simulink model "Control_Lyapunov_BarcoDiferencial"  (R2022a)
settings: Solver=VariableStepAuto  StartTime=0.0  StopTime=600  RelTol=1e-3
libraries: robotcorelib x3
settings Model: Creator=Lenovo  LastModifiedBy=Lenovo

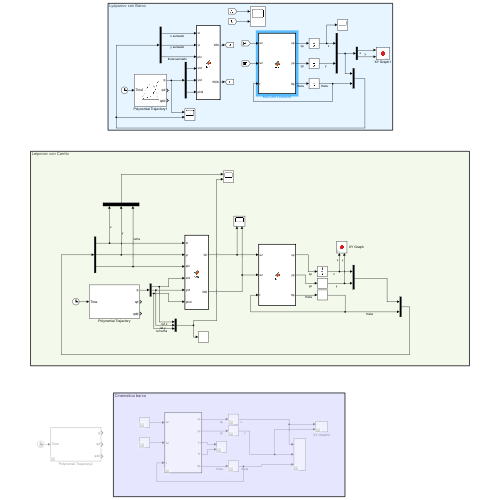
[thumbnail: Simulink's stored preview of the top-level diagram]
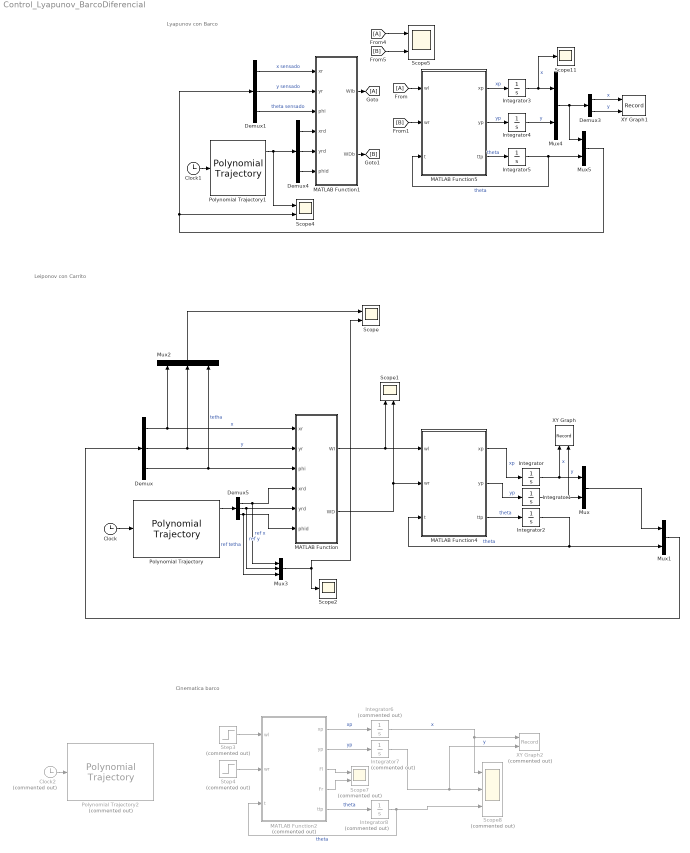
== system Control_Lyapunov_BarcoDiferencial ==
  note: Leiponov con Carrito
  note: Lyapunov con Barco
  note: Cinematica barco
  Clock : Clock
  Clock1 : Clock
  Clock2 : Clock  Commented=on
  Demux{,1,4..5} (4 alike) : Demux  Outputs=3
  Demux3 : Demux  Outputs=2
  From : From
  From4 : From
  Goto : Goto
  Integrator : Integrator  InitialCondition=0.0001
  Integrator1 : Integrator
  Integrator2 : Integrator
  Integrator3 : Integrator  InitialCondition=10
  Integrator4 : Integrator  InitialCondition=5
  Integrator5 : Integrator  InitialCondition=2.7
  Integrator6 : Integrator  Commented=on  InitialCondition=5
  Integrator7 : Integrator  Commented=on  InitialCondition=5
  Integrator8 : Integrator  Commented=on
  MATLAB Function : MATLAB Function  TreatAsAtomicUnit=on
  MATLAB Function1 : MATLAB Function  TreatAsAtomicUnit=on
  MATLAB Function2 : MATLAB Function  Commented=on  TreatAsAtomicUnit=on
  MATLAB Function4 : MATLAB Function  TreatAsAtomicUnit=on
  MATLAB Function5 : MATLAB Function  TreatAsAtomicUnit=on
  Mux{,1,4..5} (4 alike) : Mux  Inputs=2
  Mux2 : Mux  Inputs=3
  Mux3 : Mux  Inputs=3
  Polynomial Trajectory : robotcorelib/Polynomial Trajectory  WaypointSource=Internal  Waypoints=[ 0 5; 0 10; 0 1.578]  TimePoints=[ 0, 50 ]  TimeInterval=[ 1, 4 ]  Method=Cubic Polynomial  ParameterSource=Internal  VelocityBoundaryCondition=zeros( 3, 2)  AccelerationBoundaryCondition=zeros( 2, 5 )  SimulateUsing=Interpreted execution
      settings: SourceProductBaseCode=RO,NV,RR,UV
  Polynomial Trajectory1 : robotcorelib/Polynomial Trajectory  WaypointSource=Internal  Waypoints=[10 12; 5 10; 2.7 1.5]  TimePoints=[0 10]  TimeInterval=[ 1, 4 ]  Method=Cubic Polynomial  ParameterSource=Internal  VelocityBoundaryCondition=zeros( 3, 2)  AccelerationBoundaryCondition=zeros( 2, 5 )  SimulateUsing=Interpreted execution
      settings: SourceProductBaseCode=RO,NV,RR,UV
  Polynomial Trajectory2 : robotcorelib/Polynomial Trajectory  Commented=on  WaypointSource=Internal  Waypoints=[ 0 5; 0 5; 0 1.578]  TimePoints=[ 0 20 ]  TimeInterval=[ 1, 4 ]  Method=Cubic Polynomial  ParameterSource=Internal  VelocityBoundaryCondition=zeros( 3, 2)  AccelerationBoundaryCondition=zeros( 2, 5 )  SimulateUsing=Interpreted execution
      settings: SourceProductBaseCode=RO,NV,RR,UV
  Scope{,1,4..5} (4 alike) : Scope  NumInputPorts=2
  Scope11 : Scope
  Scope2 : Scope
  Scope7 : Scope  Commented=on  NumInputPorts=2
  Scope8 : Scope  Commented=on  NumInputPorts=3
  Step3 : Step  Commented=on  Time=0  After=10  SampleTime=0
  Step4 : Step  Commented=on  Time=0  After=5  SampleTime=0
  XY Graph : Record  FileSettingsInternal="{\"entries\":[{\"content\":{\"excelSettings\":{\"content\":{},\"type\":\"Streamout.ExcelSettings\"}},\"type\":\"Streamout.FileSettingStorage\",\"uuid\":\"7295fb2b-ff57-43ce-bb86-fdd5f6b61bc5\"}],\"packageUris\":[\"http://schema.mathworks.com/mf0/streamout_blocks/R2020a\"],\"version\":\"1.0\"}"  Layout=[1 1]  SignalsInternal="{\"entries\":[{\"content\":{\"signals\":[{\"content\":{\"blockPath\":[\"Diagrma_Base2/XY Graph\"],\"channel\":[],\"dimensions\":[1],\"domain\":\"Diagrma_Base2/XY Graph\",\"lineColor\":\"#a2142f\",\"plots\":[1],\"port\":1,\"sid\":[],\"signalID\":17,\"signalName\":\"x\"},\"type\":\"RecordBlkView.Signal\",\"uuid\":\"777eca82-6aae-4ff1-8555-769b58b9b1a9\"},{\"content\":{\"blockPath\":[\"Diagrma_Base2/XY Graph\"],\"channel\":[],\"dimensions\":[1],\"domain\":\"Diagrma_Base2/XY Graph\",\"lineColor\":\"#139fff\",\"plots\":[1],\"port\":2,\"sid\":[],\"signalID\":20,\"signalName\":\"y\"},\"type\":\"RecordBlkView.Signal\",\"uuid\":\"4820c845-bf9c-47bf-9568-d466896c225b\"}]},\"type\":\"RecordBlkView.InputSignals\",\"uuid\":\"f7904860-0271-4dba-87b7-ce7dfbb5efd7\"}],\"packageUris\":[\"http://schema.mathworks.com/mf0/streamout_blocks/R2020a\"],\"version\":\"1.0\"}"  VisualizationBindings="{\"xyplotplugin\":{\"info\":[{\"series\":[{\"bindingParametersList\":[{\"parameter\":\"X-Axis\",\"signalID\":17,\"signalName\":\"x\"},{\"parameter\":\"Y-Axis\",\"signalID\":20,\"signalName\":\"y\"}],\"seriesID\":12843}],\"subplotID\":1}]}}"  CompatibilityTag=XY
  XY Graph1 : Record  FileSettingsInternal="{\"entries\":[{\"content\":{\"excelSettings\":{\"content\":{},\"type\":\"Streamout.ExcelSettings\"}},\"type\":\"Streamout.FileSettingStorage\",\"uuid\":\"a2b37473-8bde-4ada-a6ad-28720db650b0\"}],\"packageUris\":[\"http://schema.mathworks.com/mf0/streamout_blocks/R2020a\"],\"version\":\"1.0\"}"  Layout=[1 1]  SignalsInternal="{\"entries\":[{\"content\":{\"signals\":[{\"content\":{\"blockPath\":[\"Diagrma_Base2/XY Graph1\"],\"channel\":[],\"dimensions\":[1],\"domain\":\"Diagrma_Base2/XY Graph1\",\"lineColor\":\"#a2142f\",\"plots\":[1],\"port\":1,\"sid\":[],\"signalID\":9,\"signalName\":\"x\"},\"type\":\"RecordBlkView.Signal\",\"uuid\":\"0c049299-8119-4ead-a456-183b3d2d228e\"},{\"content\":{\"blockPath\":[\"Diagrma_Base2/XY Graph1\"],\"channel\":[],\"dimensions\":[1],\"domain\":\"Diagrma_Base2/XY Graph1\",\"lineColor\":\"#139fff\",\"plots\":[1],\"port\":2,\"sid\":[],\"signalID\":12,\"signalName\":\"y\"},\"type\":\"RecordBlkView.Signal\",\"uuid\":\"c17ab7cf-dfc4-43cc-b6cb-2b06547cf23f\"}]},\"type\":\"RecordBlkView.InputSignals\",\"uuid\":\"baae757a-dbf7-4c06-a341-545d20dfedee\"}],\"packageUris\":[\"http://schema.mathworks.com/mf0/streamout_blocks/R2020a\"],\"version\":\"1.0\"}"  VisualizationBindings="{\"xyplotplugin\":{\"info\":[{\"series\":[{\"bindingParametersList\":[{\"parameter\":\"X-Axis\",\"signalID\":9,\"signalName\":\"x\"},{\"parameter\":\"Y-Axis\",\"signalID\":12,\"signalName\":\"y\"}],\"seriesID\":46415}],\"subplotID\":1}]}}"  CompatibilityTag=XY
  XY Graph2 : Record  Commented=on  FileSettingsInternal="{\"entries\":[{\"content\":{\"excelSettings\":{\"content\":{},\"type\":\"Streamout.ExcelSettings\"}},\"type\":\"Streamout.FileSettingStorage\",\"uuid\":\"b3166ed0-6056-44fb-bfad-bac826df8843\"}],\"packageUris\":[\"http://schema.mathworks.com/mf0/streamout_blocks/R2020a\"],\"version\":\"1.0\"}"  Layout=[1 1]  SignalsInternal="{\"entries\":[{\"content\":{\"signals\":[{\"content\":{\"blockPath\":[\"Diagrma_Base2/XY Graph2\"],\"channel\":[],\"dimensions\":[1],\"domain\":\"Diagrma_Base2/XY Graph2\",\"lineColor\":\"#a2142f\",\"plots\":[1],\"port\":1,\"sid\":[],\"signalID\":25,\"signalName\":\"x\"},\"type\":\"RecordBlkView.Signal\",\"uuid\":\"49568a3e-d36f-41cf-8f23-ccc7c9185f6e\"},{\"content\":{\"blockPath\":[\"Diagrma_Base2/XY Graph2\"],\"channel\":[],\"dimensions\":[1],\"domain\":\"Diagrma_Base2/XY Graph2\",\"lineColor\":\"#139fff\",\"plots\":[1],\"port\":2,\"sid\":[],\"signalID\":28,\"signalName\":\"y\"},\"type\":\"RecordBlkView.Signal\",\"uuid\":\"cb959886-84b1-405c-8f57-00818f683079\"}]},\"type\":\"RecordBlkView.InputSignals\",\"uuid\":\"66f7ff6e-8114-4676-a999-c205b5aca1eb\"}],\"packageUris\":[\"http://schema.mathworks.com/mf0/streamout_blocks/R2020a\"],\"version\":\"1.0\"}"  VisualizationBindings="{\"xyplotplugin\":{\"info\":[{\"series\":[{\"bindingParametersList\":[{\"parameter\":\"X-Axis\",\"signalID\":25,\"signalName\":\"x\"},{\"parameter\":\"Y-Axis\",\"signalID\":28,\"signalName\":\"y\"}],\"seriesID\":189}],\"subplotID\":1}]}}"  CompatibilityTag=XY
  wires:
  MATLAB Function/1(WI) -> Scope1/1, MATLAB Function4/1(wl)
  MATLAB Function/2(WD) -> Scope1/2, MATLAB Function4/2(wr)
  MATLAB Function4/1(xp) -> Integrator/1  "xp"
  MATLAB Function4/2(yp) -> Integrator1/1  "yp"
  MATLAB Function4/3(ttp) -> Integrator2/1  "theta"
  Mux/1 -> Mux1/1
  Demux/2 -> Mux2/2, MATLAB Function/2(yr)  "y"
  Mux2/1 -> Scope/1
  Integrator2/1 -> MATLAB Function4/3(t), Mux1/2  "theta"
  Clock/1 -> Polynomial Trajectory/1
  Mux1/1 -> Demux/1
  Integrator1/1 -> XY Graph/2, Mux/2  "y"
  Integrator/1 -> XY Graph/1, Mux/1  "x"
  Mux3/1 -> Scope2/1, Scope/2
  Demux/1 -> Mux2/1, MATLAB Function/1(xr)  "x"
  Demux/3 -> Mux2/3, MATLAB Function/3(phi)  "tetha"
  Mux5/1 -> Scope4/2, Demux1/1
  Demux1/2 -> MATLAB Function1/2(yr)  "y sensado"
  Demux3/1 -> XY Graph1/1  "x"
  Demux1/3 -> MATLAB Function1/3(phi)  "theta sensado"
  Demux1/1 -> MATLAB Function1/1(xr)  "x sensado"
  MATLAB Function5/2(yp) -> Integrator4/1  "yp"
  Integrator5/1 -> MATLAB Function5/3(t), Mux5/2  "theta"
  MATLAB Function5/3(ttp) -> Integrator5/1  "theta"
  Demux3/2 -> XY Graph1/2  "y"
  MATLAB Function5/1(xp) -> Integrator3/1  "xp"
  Integrator4/1 -> Mux4/2  "y"
  Integrator3/1 -> Scope11/1, Mux4/1  "x"
  Mux4/1 -> Demux3/1, Mux5/1
  Clock1/1 -> Polynomial Trajectory1/1
  Demux4/1 -> MATLAB Function1/4(xrd)
  Demux4/3 -> MATLAB Function1/6(phid)
  Demux4/2 -> MATLAB Function1/5(yrd)
  Integrator8/1 -> Scope8/3, MATLAB Function2/3(t)  "theta"
  Integrator6/1 -> XY Graph2/1, Scope8/1  "x"
  MATLAB Function2/5(ttp) -> Integrator8/1  "theta"
  Integrator7/1 -> XY Graph2/2, Scope8/2  "y"
  MATLAB Function2/2(yp) -> Integrator7/1  "yp"
  MATLAB Function2/1(xp) -> Integrator6/1  "xp"
  MATLAB Function2/3(Fl) -> Scope7/1
  MATLAB Function2/4(Fr) -> Scope7/2
  Step4/1 -> MATLAB Function2/2(wr)
  Step3/1 -> MATLAB Function2/1(wl)
  Polynomial Trajectory/1 -> Demux5/1
  Demux5/1 -> MATLAB Function/4(xrd), Mux3/1  "ref x"
  Demux5/2 -> Mux3/2, MATLAB Function/5(yrd)  "ref y"
  Demux5/3 -> MATLAB Function/6(phid), Mux3/3  "ref tetha"
  Clock2/1 -> Polynomial Trajectory2/1
  From4/1 -> Scope5/1
  [B] -> Scope5/2
  MATLAB Function1/1(WIb) -> Goto/1
  From/1 -> MATLAB Function5/1(wl)
  MATLAB Function1/2(WDb) -> [B]
  [B] -> MATLAB Function5/2(wr)
  Polynomial Trajectory1/1 -> Scope4/1, Demux4/1

== matlab function Control_Lyapunov_BarcoDiferencial/MATLAB Function1 ==
  data: xr input; yr input; phi input; xrd input; WIb output; WDb output; yrd input; phid input
function [WIb, WDb]  = fcn(xr, yr, phi, xrd, yrd, phid)
%------------valores barco---------
Lb = 0.87;
Db = 0.435;
K1 = 1;
K2 = 1;
q2 = 1;

% 4) Control
%a) Errores de control
l = sqrt((xrd - xr)^2 + (yrd - yr)^2);
zeta = atan2((yrd - yr), (xrd - xr)) - phi;
psi = atan2((yrd - yr), (xrd - xr)) - phid;
%b) Ley de control
u = K1 * cos(zeta) * l; % Velocidad lineal de entrada
w = K2 * zeta + (K1/zeta) * cos(zeta) * sin(zeta) * (zeta + q2 * psi); % Velocidad angular de entrada

% p -> densidad agua (kg/m^3)
p = 1000;
% r -> radio del motor
r = 0.065;
% A -> Area de la seccion transversal del motor (m^2)
A = (pi*0.065^2);
Fl = p*A*r^2;          % Fuerza de la hélice izquierda (N/s)
Fr = p*A*r^2;          % Fuerza de la hélice derecha (N/s)
%c) velocidades angulares:
% Bote
WDb = Fr*(2*u + Lb*w)/(2*Db);
WIb = Fl*(2*u - Lb*w)/(2*Db);

== matlab function Control_Lyapunov_BarcoDiferencial/MATLAB Function ==
  data: xr input; yr input; phi input; xrd input; WI output; WD output; yrd input; phid input
function [WI, WD]  = fcn(xr, yr, phi, xrd, yrd, phid)
L = 0.87;
D = 0.435;
R = 0.130;
% 2) Condiciones iniciales
% xr, yr, phi

% 3) Referencias deseadas
% xrd, yrd, phid

K1 = 1;
K2 = 1;
q2 = 1;

% 4) Control
%a) Errores de control
l = sqrt((xrd - xr)^2 + (yrd - yr)^2);
zeta = atan2((yrd - yr), (xrd - xr)) - phi;
psi = atan2((yrd - yr), (xrd - xr)) - phid;

%b) Ley de control
u = K1 * cos(zeta) * l; % Velocidad lineal de entrada
w = K2 * zeta + (K1/zeta) * cos(zeta) * sin(zeta) * (zeta + q2 * psi); % Velocidad angular de entrada

%c) velocidades angulares:

% WI = (τ/J)-((Fw + Fp)*d/(2*J));
% WD = (τ/J)-((Fw + Fp)*d/(2*J));

%WD = (2*u + L*w)/(2*D);
%WI = (2*u - L*w)/(2*D);

WD = (u + w*(L/2))/R;
WI = (u - w*(L/2))/R;

== matlab function Control_Lyapunov_BarcoDiferencial/MATLAB Function4 ==
  data: wl input; xp output; wr input; yp output; ttp output; t input
function [xp,yp,ttp] = fcn(wl,wr,t)
R = 0.06;
L = 0.6;

W = [wr; wl];
M = [(R*cos(t)/2) (R*cos(t)/2);
     (R*sin(t)/2) (R*sin(t)/2);
      R/L          -R/L] * W;

xp = M(1,1);
yp = M(2,1);
ttp = M(3,1);

== matlab function Control_Lyapunov_BarcoDiferencial/MATLAB Function2 ==
  data: wl input; xp output; wr input; yp output; Fl output; Fr output; ttp output; t input
function [xp,yp, Fl,Fr,ttp] = fcn(wl,wr,t)
psi=t;
% Parámetros del barco
m = 36.38;           % masa total del barco (kg)
Iz = 16485605.66/1000000;          % momento de inercia del barco alrededor del eje vertical (kg*m^2)
cg = 0.05;             % distancia desde el centro del barco hasta el centro de masa (m)
d = 0.435;            % distancia entre el centro del barco y el eje de la hélice (m)
L = 0.87;             % distancia entre las hélices del barco (m)
D = 1.7973e+02;       % resistencia hidrodinámica ejercida por el agua sobre el casco del barco (N)

% Velocidades de las hélices

% p -> densidad agua (kg/m^3)
p = 1000;
% r -> radio del motor
r = 0.065;
% A -> Area de la seccion transversal del motor (m^2)
A = (pi*0.065^2);

% v -> velocidad lineal (m/s)
% w -> velocidad angular

% v = w*r
% F = p*A*v^2 (N)
g = 9.81;
%V = 0.06441900128;
%pm = m/V;
%F = p*V*g*m/((1-p)/pm);
Fl = p*A*(wl*r)^2          % Fuerza de la hélice izquierda (N/s)
Fr = p*A*(wr*r)^2          % Fuerza de la hélice derecha (N/s)

% Ecuación de cinemática
A = [cos(psi) 0; 
     sin(psi) 0; 
     0 1];
B1 = [1/m*(Fl + Fr - D); 
      0];
B2 = [0; 
      0; 
      1/Iz*(Fr - Fl)*(d/2 - cg)];
M = A * B1 + B2;

xp = M(1,1);
yp = M(2,1);
ttp = M(3,1);

% R = 0.130;
% L = 87;
% 
% W = [wr;
%     wl];
% M = [(R*cos(t)/2) (R*cos(t)/2);
%      (R*sin(t)/2) (R*sin(t)/2);
%       R/L          -R/L] * W;
% 
% xp = M(1,1);
% yp = M(2,1);
% ttp = M(3,1);

== matlab function Control_Lyapunov_BarcoDiferencial/MATLAB Function5 ==
  data: wl input; xp output; wr input; yp output; ttp output; t input
function [xp,yp,ttp] = fcn(wl,wr,t)
R = 0.130;
L = 0.87;

W = [wr; wl];
M = [(R*cos(t)/2) (R*cos(t)/2);
     (R*sin(t)/2) (R*sin(t)/2);
      R/L          -R/L] * W;

xp = M(1,1);
yp = M(2,1);
ttp = M(3,1);
